simulink model "ballAndBeamModel"  (R2021b)
settings: Solver=ode5  StartTime=0.0  StopTime=inf  RelTol=1e-3
libraries: sldrtlib x1
settings Model: Creator=sansh  LastModifiedBy=matij
settings SolverCC: AlgebraicLoopSolver=TrustRegion
settings DataIOCC: ReturnWorkspaceOutputs=off
settings DebuggingCC: SFMachineParentedDataDiag=warning  ArithmeticOperatorsInVariantConditions=warning
settings SFSimCC: SimUseLocalCustomCode=off  CustomCodeUndefinedFunction=UseInterfaceOnly
settings RTWCC: Description=Simulink Desktop Real-Time  SystemTargetFile=sldrt.tlc  TemplateMakefile=sldrt.tmf  RTWUseLocalCustomCode=off  RTWCompilerOptimization=on
settings CodeAppCC: MaxIdLength=95  StateflowObjectComments=on
settings SimulinkDesktopRealTimeCC: TargetPreCompLibLocation=C:\Program Files\MATLAB\R2021b\toolbox\sldrt\lib\win64

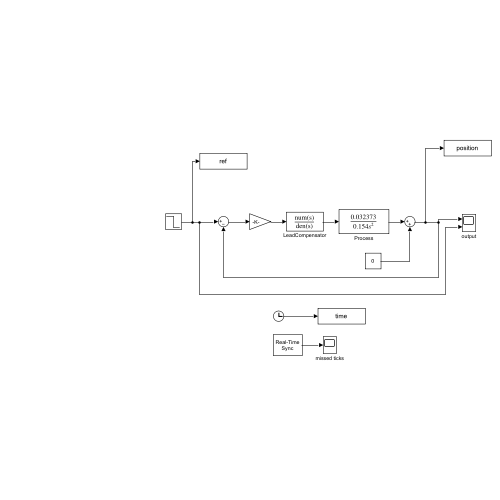
[thumbnail: Simulink's stored preview of the top-level diagram]
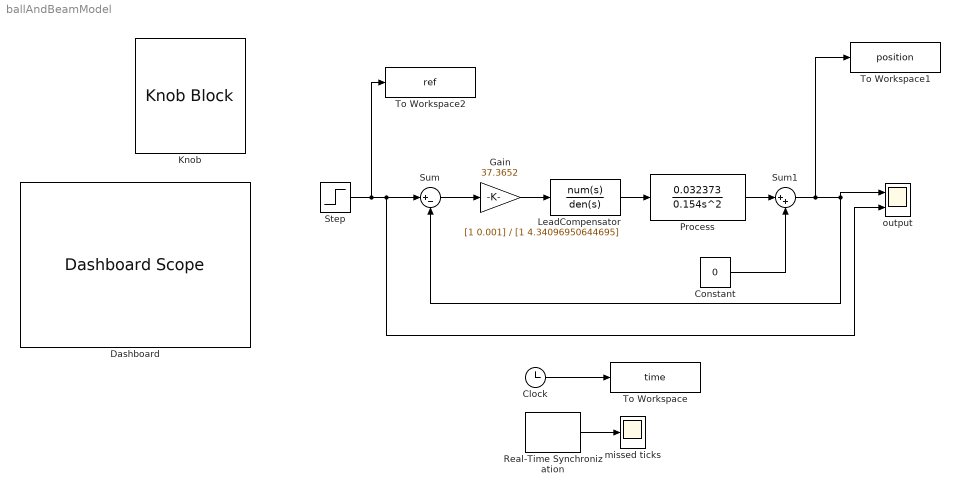
== system ballAndBeamModel ==
  Clock : Clock
  Constant : Constant  Value=0
  Dashboard : DashboardScope  Ymin=0  Ymax=1.2  ScaleAtStop=off  UpdateMode=Scroll
  Gain : Gain  Gain=37.3652
  Knob : KnobBlock  ScaleMin=-1  ScaleMax=1
  LeadCompensator : TransferFcn  Numerator=[1 0.001]  Denominator=[1 4.34096950644695]
  Process : TransferFcn  Numerator=[0 0 0.032373]  Denominator=[0.154 0 0]
  Real-Time Synchronization : sldrtlib/Real-Time Synchronization  SampleTime=0.01  MaxMissedTicks=inf  ShowMissedTicks=on  YieldWhenWaiting=off
  Step : Step  Time=0  After=-0.29046  SampleTime=0
  Sum : Sum  Inputs=|+-
  Sum1 : Sum  Inputs=|++
  To Workspace : ToWorkspace  VariableName=time  SaveFormat=Structure With Time  SampleTime=-1
  To Workspace1 : ToWorkspace  VariableName=position  SaveFormat=Structure With Time  SampleTime=-1
  To Workspace2 : ToWorkspace  VariableName=ref  SaveFormat=Structure With Time  SampleTime=-1
  missed ticks : Scope
  output : Scope  NumInputPorts=2
  wires:
  Gain/1 -> LeadCompensator/1
  Sum/1 -> Gain/1
  Clock/1 -> To Workspace/1
  LeadCompensator/1 -> Process/1
  Process/1 -> Sum1/1
  Constant/1 -> Sum1/2
  Sum1/1 -> To Workspace1/1, output/1, Sum/2
  Real-Time Synchronization/1 -> missed ticks/1
  Step/1 -> To Workspace2/1, output/2, Sum/1
